simulink library "partitionedLifitngBdyForces_ul"  (R2018b)
settings: Solver=VariableStepAuto  StartTime=0.0  StopTime=10.0  RelTol=1e-3
values from neighbouring files (symbols this model uses):
  env = ENV.environment    [partitionedLifitngBdy_ts.m]
  vhcl = PLT.vehicle    [partitionedLifitngBdy_ts.m]
libraries: vrlib x3, eulAng2RotMat_ul x1, alphaBeta_ul x1, dynamicPressure_ul x1, surfaceCoefficients_ul x1, vectorDirection x1
settings Model: Creator=mcobb  LastModifiedBy=asiddiq2

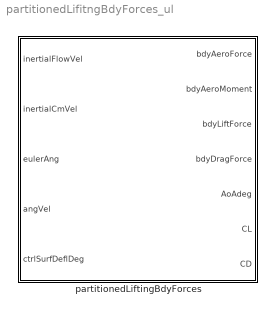
== system partitionedLifitngBdyForces_ul ==
  partitionedLiftingBdyForces : Subsystem  mask{rhoFluid=env.fluidDensity.Value, aeroCenterPos=vhcl.fluidMomentArms.Value, fluidRefArea=vhcl.fluidRefArea.Value, FluidStruct=vhcl.fluidCoeffData}
      mask prompts: rhoFluid "Fluid density"; aeroCenterPos "Fluid dynamic center position vectors"; fluidRefArea "Fluid dynamic reference area"; FluidStruct "Fluid dynamic data structure"
      mask TypeOptions rhoFluid: dynamicPressure/rhoFluid
      mask DialogControl ParameterGroupVar Prompt: Environment
      mask DialogControl Container3 Prompt: Fluid dynamic reference values
      mask DialogControl Container3_copy Prompt: Fluid dynamic coefficient data

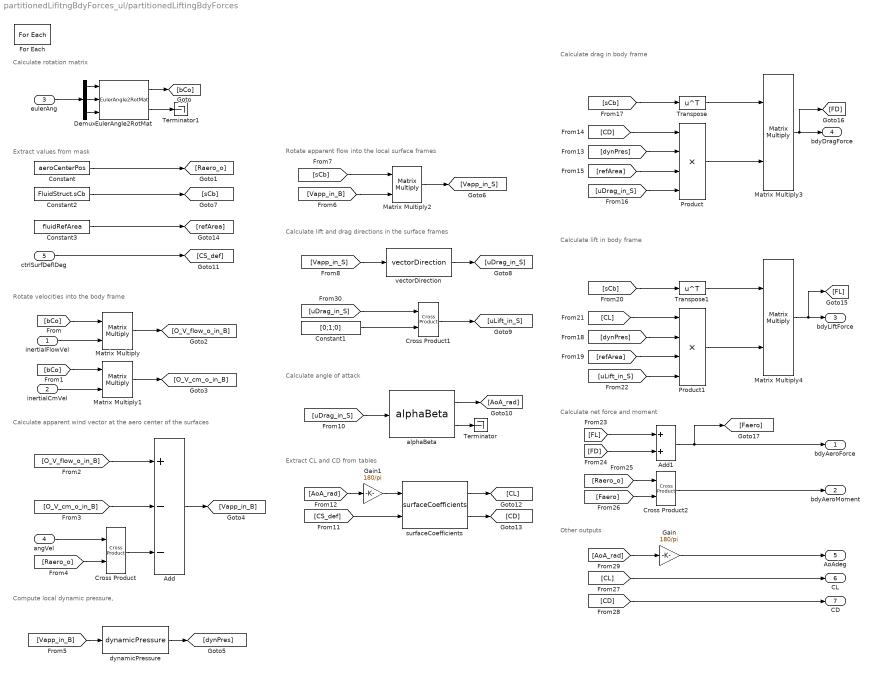
== system partitionedLifitngBdyForces_ul/partitionedLiftingBdyForces ==
  note: Calculate angle of attack
  note: Calculate lift and drag directions in the surface frames
  note: Rotate apparent flow into the local surface frames
  note: Rotate velocities into the body frame
  note: Extract values from mask
  note: Calculate rotation matrix
  note: Calculate net force and moment
  note: Compute local dynamic pressure,
  note: Calculate drag in body frame
  note: Calculate apparent wind vector at the aero center of the surfaces
  note: Extract CL and CD from tables
  note: Calculate lift in body frame
  note: Other outputs
  inertialFlowVel : Inport  PortDimensions=[3,1]
  inertialCmVel : Inport  Port=2  PortDimensions=[3,1]
  eulerAng : Inport  Port=3  PortDimensions=[3,1]
  angVel : Inport  Port=4  PortDimensions=[3,1]
  ctrlSurfDeflDeg : Inport  Port=5  PortDimensions=[1,1]  Partition=on  PartitionDimension=1  PartitionWidth=1  PartitionOffset=0
  Add : Sum  Inputs=+--
  Add1 : Sum
  Constant : Constant  Value=aeroCenterPos  VectorParams1D=off
  Constant1 : Constant  Value=[0;1;0]  VectorParams1D=off
  Constant2 : Constant  Value=FluidStruct.sCb  VectorParams1D=off
  Constant3 : Constant  Value=fluidRefArea  VectorParams1D=off
  Cross Product : vrlib/Utilities/Cross Product
      settings: SourceProductBaseCode=VR
  Cross Product1 : vrlib/Utilities/Cross Product
      settings: SourceProductBaseCode=VR
  Cross Product2 : vrlib/Utilities/Cross Product
      settings: SourceProductBaseCode=VR
  Demux : Demux  Outputs=3
  EulerAngle2RotMat : eulAng2RotMat_ul/EulerAngle2RotMat  SystemSampleTime=-1
  For Each : ForEach  DisableCoverage=on  IterateSubsysMaskParameter=off,on,off,on  SubsysMaskParameterIterationDimension=1,2,1,2  IndexMode=One-based
  Gain : Gain  Gain=180/pi
  Gain1 : Gain  Gain=180/pi
  Matrix Multiply{,1..4} (5 alike) : Product  Multiplication=Matrix(*)
  Product : Product  Inputs=4
  Product1 : Product  Inputs=4
  Terminator : Terminator
  Terminator1 : Terminator
  Transpose : Math  Operator=transpose  SaturateOnIntegerOverflow=on
  Transpose1 : Math  Operator=transpose  SaturateOnIntegerOverflow=on
  alphaBeta : alphaBeta_ul/alphaBeta  SystemSampleTime=-1
  dynamicPressure : dynamicPressure_ul/dynamicPressure  rhoFluid=rhoFluid
  surfaceCoefficients : surfaceCoefficients_ul/surfaceCoefficients  CLvals=FluidStruct.CL  CDvals=FluidStruct.CD  alphaVals=FluidStruct.alpha  GainCL=FluidStruct.GainCL  GainCD=FluidStruct.GainCD
  vectorDirection : vectorDirection/vectorDirection  SystemSampleTime=-1
  bdyAeroForce : Outport  PortDimensions=[3,1]  ConcatenationDimension=2
  bdyAeroMoment : Outport  Port=2  PortDimensions=[3,1]  ConcatenationDimension=2
  bdyLiftForce : Outport  Port=3  PortDimensions=[3,1]  ConcatenationDimension=2
  bdyDragForce : Outport  Port=4  PortDimensions=[3,1]  ConcatenationDimension=2
  AoAdeg : Outport  Port=5  PortDimensions=[1,1]  ConcatenationDimension=2
  CL : Outport  Port=6  PortDimensions=[1,1]  ConcatenationDimension=2
  CD : Outport  Port=7  PortDimensions=[1,1]  ConcatenationDimension=2
  wires:
  Add/1 -> [Vapp_in_B]
  [uDrag_in_S] -> alphaBeta/1
  alphaBeta/2 -> Terminator/1
  dynamicPressure/1 -> [dynPres]
  [CS_def] -> surfaceCoefficients/2
  eulerAng/1 -> Demux/1
  Demux/1 -> EulerAngle2RotMat/1
  Demux/2 -> EulerAngle2RotMat/2
  Demux/3 -> EulerAngle2RotMat/3
  EulerAngle2RotMat/1 -> [bCo]
  EulerAngle2RotMat/2 -> Terminator1/1
  Constant/1 -> [Raero_o]
  [bCo] -> Matrix Multiply/1
  inertialFlowVel/1 -> Matrix Multiply/2
  Matrix Multiply/1 -> [O_V_flow_o_in_B]
  [bCo] -> Matrix Multiply1/1
  Matrix Multiply1/1 -> [O_V_cm_o_in_B]
  inertialCmVel/1 -> Matrix Multiply1/2
  [O_V_flow_o_in_B] -> Add/1
  [O_V_cm_o_in_B] -> Add/2
  Cross Product/1 -> Add/3
  angVel/1 -> Cross Product/1
  [Raero_o] -> Cross Product/2
  [Vapp_in_B] -> dynamicPressure/1
  [Vapp_in_B] -> Matrix Multiply2/2
  [sCb] -> Matrix Multiply2/1
  Matrix Multiply2/1 -> [Vapp_in_S]
  Constant2/1 -> [sCb]
  [Vapp_in_S] -> vectorDirection/1
  vectorDirection/1 -> [uDrag_in_S]
  Cross Product1/1 -> [uLift_in_S]
  alphaBeta/1 -> [AoA_rad]
  ctrlSurfDeflDeg/1 -> [CS_def]
  surfaceCoefficients/1 -> [CL]
  surfaceCoefficients/2 -> [CD]
  [uDrag_in_S] -> Product/4
  [refArea] -> Product/3
  [dynPres] -> Product/2
  [CD] -> Product/1
  Product/1 -> Matrix Multiply3/2
  [sCb] -> Transpose/1
  Transpose/1 -> Matrix Multiply3/1
  Matrix Multiply3/1 -> [FD], bdyDragForce/1
  [CL] -> Product1/1
  [refArea] -> Product1/3
  Transpose1/1 -> Matrix Multiply4/1
  [dynPres] -> Product1/2
  [uLift_in_S] -> Product1/4
  Product1/1 -> Matrix Multiply4/2
  [sCb] -> Transpose1/1
  Matrix Multiply4/1 -> [FL], bdyLiftForce/1
  [FL] -> Add1/1
  [FD] -> Add1/2
  Add1/1 -> [Faero], bdyAeroForce/1
  [Raero_o] -> Cross Product2/1
  [Faero] -> Cross Product2/2
  Cross Product2/1 -> bdyAeroMoment/1
  [AoA_rad] -> Gain/1
  Gain/1 -> AoAdeg/1
  [CL] -> CL/1
  [CD] -> CD/1
  Gain1/1 -> surfaceCoefficients/1
  [AoA_rad] -> Gain1/1
  Constant3/1 -> [refArea]
  [uDrag_in_S] -> Cross Product1/1
  Constant1/1 -> Cross Product1/2
